simulink model "Practica_1_simulink"  (R2024a)
settings: Solver=VariableStepAuto  StartTime=0.0  StopTime=10.0  RelTol=1e-3
settings Model: Creator=christian  LastModifiedBy=christian

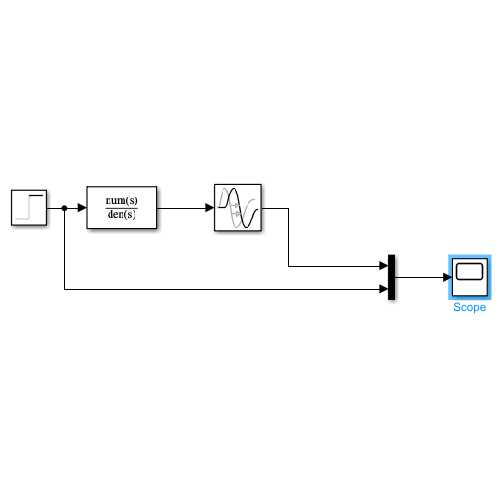
[thumbnail: Simulink's stored preview of the top-level diagram]
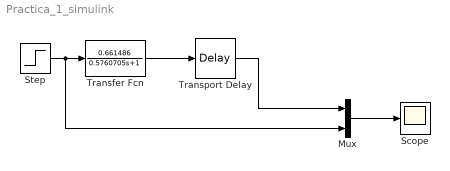
== system Practica_1_simulink ==
  Mux : Mux  Inputs=2
  Scope : Scope
  Step : Step  After=1.5  SampleTime=0
  Transfer Fcn : TransferFcn  Numerator=[0.661486]  Denominator=[0.5760705 1]
  Transport Delay : TransportDelay  DelayTime=0.4529695
  wires:
  Mux/1 -> Scope/1
  Step/1 -> Mux/2, Transfer Fcn/1
  Transfer Fcn/1 -> Transport Delay/1
  Transport Delay/1 -> Mux/1
